simulink model "rlQuadrupedRobot"  (R2020a)
settings: Solver=ode23tb  StartTime=0.0  StopTime=Tf  RelTol=1e-3  EnableMultiTasking=on
undefined symbols (not defined in the file or in its folder): Extr_Data_LinkEndHole, Extr_Data_Mesh, friction_force_max, g, ground, h_final, hip_eq_angle, init_ang_FL, init_ang_FR, init_ang_RL, init_ang_RR, joint, knee_eq_angle, l1, l2, L_back, M, m1, m2, mu_kinetic, mu_static, normal_force_max, pitch_max, q_hip_max, q_hip_min, q_knee_max, q_knee_min, roll_max, Tf, Ts, u_max, v_thres, vx_max, vy_max, vz_max, w_max, X, Y, y_max, y_min, yaw_max, Z, z_max
libraries: sm_lib x145, nesl_utility x87, simulink x12, rllib x1
(part 8 of 8)

== system rlQuadrupedRobot/Quadruped Robot/Leg RL/Contact Forces Model/Sphere to Plane Force/Forces/Ff/SlipVel ==
  wx : Inport
  wy : Inport  Port=2
  vx : Inport  Port=3
  vy : Inport  Port=4
  Fx1 : Constant  Value=sphere_rad
  Math Function : Math  Operator=square  SignedPower=on  SaturateOnIntegerOverflow=on
  Math Function1 : Math  Operator=square  SignedPower=on  SaturateOnIntegerOverflow=on
  Product3 : Product
  Product4 : Product
  Sqrt : Sqrt  SaturateOnIntegerOverflow=on
  Sum1 : Sum  Inputs=|++
  Sum2 : Sum  Inputs=|-+
  Sum3 : Sum  Inputs=|++
  Trigonometric Function : Trigonometry  Operator=atan2
  vabs : Outport  VectorParamsAs1DForOutWhenUnconnected=off
  alpha : Outport  Port=2  VectorParamsAs1DForOutWhenUnconnected=off
  wires:
  wx/1 -> Product3/1
  Product3/1 -> Sum1/1
  wy/1 -> Product4/2
  vx/1 -> Sum2/2
  Fx1/1 -> Product3/2, Product4/1
  vy/1 -> Sum1/2
  Product4/1 -> Sum2/1
  Trigonometric Function/1 -> alpha/1
  Sqrt/1 -> vabs/1
  Sum3/1 -> Sqrt/1
  Math Function/1 -> Sum3/1
  Math Function1/1 -> Sum3/2
  Sum1/1 -> Trigonometric Function/1, Math Function/1  "slipy"
  Sum2/1 -> Trigonometric Function/2, Math Function1/1  "slipx"

== system rlQuadrupedRobot/Quadruped Robot/Leg RL/Contact Forces Model/Sphere to Plane Force/Forces/Force Law/Custom ==
  note: Implement your own custom force law in this subsystem.
      | To use it in the contact force models,
      | set the parameter "Force Law" to "Custom".
  Pen : Inport
  Pen Vel : Inport  Port=2
  Abs : Abs  ZeroCross=off
  Gain1 : Gain  Gain=k_pen  Multiplication=Matrix(K*u)  SaturateOnIntegerOverflow=on  OutDataTypeStr=Inherit: Same as input  ParamDataTypeStr=Inherit: Same as input
  Gain2 : Gain  Gain=-b_penvel  Multiplication=Matrix(K*u)  SaturateOnIntegerOverflow=on  OutDataTypeStr=Inherit: Same as input  ParamDataTypeStr=Inherit: Same as input
  Product : Product  RndMeth=Zero
  Saturation : Saturate  UpperLimit=Inf  LowerLimit=0  ZeroCross=off
  Sign : Signum  ZeroCross=off
  Spr F : Outport  VectorParamsAs1DForOutWhenUnconnected=off
  Damp F : Outport  Port=2  VectorParamsAs1DForOutWhenUnconnected=off
  wires:
  Saturation/1 -> Gain2/1
  Pen/1 -> Sign/1, Gain1/1  "Penetration"
  Abs/1 -> Product/1  "Damping_Force_Enable"
  Product/1 -> Damp F/1  "Damping_Force"
  Sign/1 -> Abs/1
  Pen Vel/1 -> Saturation/1  "Pen Vel"
  Gain2/1 -> Product/2  "Damping_Force"
  Gain1/1 -> Spr F/1  "Stiffness_Force"

== system rlQuadrupedRobot/Quadruped Robot/Leg RL/Contact Forces Model/Sphere to Plane Force/Forces/Force Law/Linear ==
  Pen : Inport
  Pen Vel : Inport  Port=2
  Abs : Abs  ZeroCross=off
  Gain1 : Gain  Gain=k_pen  Multiplication=Matrix(K*u)  SaturateOnIntegerOverflow=on  OutDataTypeStr=Inherit: Same as input  ParamDataTypeStr=Inherit: Same as input
  Gain2 : Gain  Gain=-b_penvel  Multiplication=Matrix(K*u)  SaturateOnIntegerOverflow=on  OutDataTypeStr=Inherit: Same as input  ParamDataTypeStr=Inherit: Same as input
  Product : Product  RndMeth=Zero
  Saturation : Saturate  UpperLimit=Inf  LowerLimit=0  ZeroCross=off
  Sign : Signum  ZeroCross=off
  Spr F : Outport  VectorParamsAs1DForOutWhenUnconnected=off
  Damp F : Outport  Port=2  VectorParamsAs1DForOutWhenUnconnected=off
  wires:
  Saturation/1 -> Gain2/1
  Pen/1 -> Sign/1, Gain1/1  "Penetration"
  Abs/1 -> Product/1  "Damping_Force_Enable"
  Product/1 -> Damp F/1  "Damping_Force"
  Sign/1 -> Abs/1
  Pen Vel/1 -> Saturation/1  "Pen Vel"
  Gain2/1 -> Product/2  "Damping_Force"
  Gain1/1 -> Spr F/1  "Stiffness_Force"

== system rlQuadrupedRobot/Quadruped Robot/Leg RL/Contact Forces Model/Sphere to Plane Force/Forces/Force Law/Nonlinear ==
  Pen : Inport
  Pen Vel : Inport  Port=2
  Constant : Constant  Value=pen_exp
  Gain1 : Gain  Gain=k_pen  Multiplication=Matrix(K*u)  SaturateOnIntegerOverflow=on  OutDataTypeStr=Inherit: Same as input  ParamDataTypeStr=Inherit: Same as input
  Gain2 : Gain  Gain=-b_penvel  Multiplication=Matrix(K*u)  SaturateOnIntegerOverflow=on  OutDataTypeStr=Inherit: Same as input  ParamDataTypeStr=Inherit: Same as input
  Math Function : Math  Operator=pow  SignedPower=on  SaturateOnIntegerOverflow=on
  Product1 : Product  RndMeth=Zero
  Saturation : Saturate  UpperLimit=Inf  LowerLimit=0  ZeroCross=off
  Smoothstep : Subsystem  mask{min_out=0, max_out=1, step_start=0, step_finish=pen_full_damping}
      mask prompts: min_out "Minimum output"; max_out "Maximum output"; step_start "Start Step"; step_finish "Finish Step"
  Spr F : Outport  VectorParamsAs1DForOutWhenUnconnected=off
  Damp F : Outport  Port=2  VectorParamsAs1DForOutWhenUnconnected=off
  wires:
  Saturation/1 -> Gain2/1
  Product1/1 -> Damp F/1
  Smoothstep/1(Out1) -> Product1/1  "Damping_Enable"
  Gain2/1 -> Product1/2  "Damping_Force"
  Constant/1 -> Math Function/2
  Math Function/1 -> Gain1/1
  Pen/1 -> Math Function/1, Smoothstep/1(In1)  "Penetration"
  Pen Vel/1 -> Saturation/1  "Penetration_Velocity"
  Gain1/1 -> Spr F/1  "Stiffness_Force"

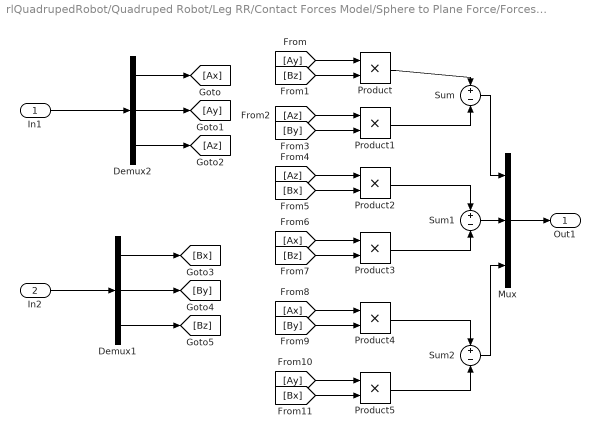
== system rlQuadrupedRobot/Quadruped Robot/Leg RR/Contact Forces Model/Sphere to Plane Force/Forces/Ff/Cross Product ==
  In1 : Inport
  In2 : Inport  Port=2
  Demux1 : Demux  Outputs=3
  Demux2 : Demux  Outputs=3
  Mux : Mux  Inputs=3
  Product{,1..5} (6 alike) : Product
  Sum : Sum  Inputs=+|-
  Sum1 : Sum  Inputs=+|-
  Sum2 : Sum  Inputs=+|-
  Out1 : Outport  VectorParamsAs1DForOutWhenUnconnected=off
  wires:
  In2/1 -> Demux1/1
  Mux/1 -> Out1/1
  Product1/1 -> Sum/2
  Product/1 -> Sum/1
  Product2/1 -> Sum1/1
  Product3/1 -> Sum1/2
  Product4/1 -> Sum2/1
  Product5/1 -> Sum2/2
  Sum1/1 -> Mux/2
  Sum/1 -> Mux/1
  Sum2/1 -> Mux/3
  In1/1 -> Demux2/1
  Demux2/1 -> [Ax]
  Demux2/2 -> [Ay]
  Demux2/3 -> [Az]
  Demux1/1 -> [Bx]
  Demux1/2 -> [By]
  Demux1/3 -> [Bz]
  [Ay] -> Product/1
  [Bz] -> Product/2
  [Az] -> Product1/1
  [By] -> Product1/2
  [Az] -> Product2/1
  [Bx] -> Product2/2
  [Ax] -> Product3/1
  [Bz] -> Product3/2
  [Ax] -> Product4/1
  [By] -> Product4/2
  [Ay] -> Product5/1
  [Bx] -> Product5/2

== system rlQuadrupedRobot/Quadruped Robot/Leg RR/Contact Forces Model/Sphere to Plane Force/Forces/Ff/Friction Law ==
  note: 1) Only subsystems can be added as variant choices at this level
      | 2) Blocks cannot be connected at this level as connectivity is
      | automatically determined at simulation, based on the active variant
  Fn : Inport
  v : Inport  Port=2
  None : Subsystem  VariantControl=None  mask(No Friction){}
      mask help: Friction Force = 0
  "Stick-Slip C " : Subsystem  VariantControl=Stick_Slip_C  mask(Stick-Slip Friction, Continuous){muk=mu_kinetic, mus=mu_static, vth=v_thr}
      mask prompts: muk "Coefficient of Kinetic Friction"; mus "Coefficient of Static Friction"; vth "Velocity Threshold"
      mask help: Implements a continuous stick-slip friction model. Smaller velocity threshold is closer to reality but results in a numerically stiffer system.
  Ff : Outport  VectorParamsAs1DForOutWhenUnconnected=off

== system rlQuadrupedRobot/Quadruped Robot/Leg RR/Contact Forces Model/Sphere to Plane Force/Forces/Ff/SlipVel ==
  wx : Inport
  wy : Inport  Port=2
  vx : Inport  Port=3
  vy : Inport  Port=4
  Fx1 : Constant  Value=sphere_rad
  Math Function : Math  Operator=square  SignedPower=on  SaturateOnIntegerOverflow=on
  Math Function1 : Math  Operator=square  SignedPower=on  SaturateOnIntegerOverflow=on
  Product3 : Product
  Product4 : Product
  Sqrt : Sqrt  SaturateOnIntegerOverflow=on
  Sum1 : Sum  Inputs=|++
  Sum2 : Sum  Inputs=|-+
  Sum3 : Sum  Inputs=|++
  Trigonometric Function : Trigonometry  Operator=atan2
  vabs : Outport  VectorParamsAs1DForOutWhenUnconnected=off
  alpha : Outport  Port=2  VectorParamsAs1DForOutWhenUnconnected=off
  wires:
  wx/1 -> Product3/1
  Product3/1 -> Sum1/1
  wy/1 -> Product4/2
  vx/1 -> Sum2/2
  Fx1/1 -> Product3/2, Product4/1
  vy/1 -> Sum1/2
  Product4/1 -> Sum2/1
  Trigonometric Function/1 -> alpha/1
  Sqrt/1 -> vabs/1
  Sum3/1 -> Sqrt/1
  Math Function/1 -> Sum3/1
  Math Function1/1 -> Sum3/2
  Sum1/1 -> Trigonometric Function/1, Math Function/1  "slipy"
  Sum2/1 -> Trigonometric Function/2, Math Function1/1  "slipx"

== system rlQuadrupedRobot/Quadruped Robot/Leg RR/Contact Forces Model/Sphere to Plane Force/Forces/Force Law/Custom ==
  note: Implement your own custom force law in this subsystem.
      | To use it in the contact force models,
      | set the parameter "Force Law" to "Custom".
  Pen : Inport
  Pen Vel : Inport  Port=2
  Abs : Abs  ZeroCross=off
  Gain1 : Gain  Gain=k_pen  Multiplication=Matrix(K*u)  SaturateOnIntegerOverflow=on  OutDataTypeStr=Inherit: Same as input  ParamDataTypeStr=Inherit: Same as input
  Gain2 : Gain  Gain=-b_penvel  Multiplication=Matrix(K*u)  SaturateOnIntegerOverflow=on  OutDataTypeStr=Inherit: Same as input  ParamDataTypeStr=Inherit: Same as input
  Product : Product  RndMeth=Zero
  Saturation : Saturate  UpperLimit=Inf  LowerLimit=0  ZeroCross=off
  Sign : Signum  ZeroCross=off
  Spr F : Outport  VectorParamsAs1DForOutWhenUnconnected=off
  Damp F : Outport  Port=2  VectorParamsAs1DForOutWhenUnconnected=off
  wires:
  Saturation/1 -> Gain2/1
  Pen/1 -> Sign/1, Gain1/1  "Penetration"
  Abs/1 -> Product/1  "Damping_Force_Enable"
  Product/1 -> Damp F/1  "Damping_Force"
  Sign/1 -> Abs/1
  Pen Vel/1 -> Saturation/1  "Pen Vel"
  Gain2/1 -> Product/2  "Damping_Force"
  Gain1/1 -> Spr F/1  "Stiffness_Force"

== system rlQuadrupedRobot/Quadruped Robot/Leg RR/Contact Forces Model/Sphere to Plane Force/Forces/Force Law/Linear ==
  Pen : Inport
  Pen Vel : Inport  Port=2
  Abs : Abs  ZeroCross=off
  Gain1 : Gain  Gain=k_pen  Multiplication=Matrix(K*u)  SaturateOnIntegerOverflow=on  OutDataTypeStr=Inherit: Same as input  ParamDataTypeStr=Inherit: Same as input
  Gain2 : Gain  Gain=-b_penvel  Multiplication=Matrix(K*u)  SaturateOnIntegerOverflow=on  OutDataTypeStr=Inherit: Same as input  ParamDataTypeStr=Inherit: Same as input
  Product : Product  RndMeth=Zero
  Saturation : Saturate  UpperLimit=Inf  LowerLimit=0  ZeroCross=off
  Sign : Signum  ZeroCross=off
  Spr F : Outport  VectorParamsAs1DForOutWhenUnconnected=off
  Damp F : Outport  Port=2  VectorParamsAs1DForOutWhenUnconnected=off
  wires:
  Saturation/1 -> Gain2/1
  Pen/1 -> Sign/1, Gain1/1  "Penetration"
  Abs/1 -> Product/1  "Damping_Force_Enable"
  Product/1 -> Damp F/1  "Damping_Force"
  Sign/1 -> Abs/1
  Pen Vel/1 -> Saturation/1  "Pen Vel"
  Gain2/1 -> Product/2  "Damping_Force"
  Gain1/1 -> Spr F/1  "Stiffness_Force"

== system rlQuadrupedRobot/Quadruped Robot/Leg RR/Contact Forces Model/Sphere to Plane Force/Forces/Force Law/Nonlinear ==
  Pen : Inport
  Pen Vel : Inport  Port=2
  Constant : Constant  Value=pen_exp
  Gain1 : Gain  Gain=k_pen  Multiplication=Matrix(K*u)  SaturateOnIntegerOverflow=on  OutDataTypeStr=Inherit: Same as input  ParamDataTypeStr=Inherit: Same as input
  Gain2 : Gain  Gain=-b_penvel  Multiplication=Matrix(K*u)  SaturateOnIntegerOverflow=on  OutDataTypeStr=Inherit: Same as input  ParamDataTypeStr=Inherit: Same as input
  Math Function : Math  Operator=pow  SignedPower=on  SaturateOnIntegerOverflow=on
  Product1 : Product  RndMeth=Zero
  Saturation : Saturate  UpperLimit=Inf  LowerLimit=0  ZeroCross=off
  Smoothstep : Subsystem  mask{min_out=0, max_out=1, step_start=0, step_finish=pen_full_damping}
      mask prompts: min_out "Minimum output"; max_out "Maximum output"; step_start "Start Step"; step_finish "Finish Step"
  Spr F : Outport  VectorParamsAs1DForOutWhenUnconnected=off
  Damp F : Outport  Port=2  VectorParamsAs1DForOutWhenUnconnected=off
  wires:
  Saturation/1 -> Gain2/1
  Product1/1 -> Damp F/1
  Smoothstep/1(Out1) -> Product1/1  "Damping_Enable"
  Gain2/1 -> Product1/2  "Damping_Force"
  Constant/1 -> Math Function/2
  Math Function/1 -> Gain1/1
  Pen/1 -> Math Function/1, Smoothstep/1(In1)  "Penetration"
  Pen Vel/1 -> Saturation/1  "Penetration_Velocity"
  Gain1/1 -> Spr F/1  "Stiffness_Force"

== system rlQuadrupedRobot/Quadruped Robot/Leg FL/Contact Forces Model/Sphere to Plane Force/Forces/Ff/Friction Law/None ==
  Fn : Inport
  v : Inport  Port=2
  Constant : Constant  Value=0
  Terminator : Terminator
  Terminator1 : Terminator
  Ff : Outport  VectorParamsAs1DForOutWhenUnconnected=off
  wires:
  Constant/1 -> Ff/1  "Friction_Force"
  v/1 -> Terminator/1  "Velocity"
  Fn/1 -> Terminator1/1  "Normal_Force"

== system rlQuadrupedRobot/Quadruped Robot/Leg FL/Contact Forces Model/Sphere to Plane Force/Forces/Ff/Friction Law/Stick-Slip C  ==
  Fn : Inport
  v : Inport  Port=2
  Coefficient of Friction vs Velocity : Lookup_n-D  NumberOfTableDimensions=1  BreakpointsForDimension1=[-3 -1.5 -1 1 1.5 3]*vth  Table="[-muk -muk -mus mus  muk muk]"  InternalRulePriority=Speed  InputSameDT=on
  Gain2 : Gain  Multiplication=Matrix(K*u)  SaturateOnIntegerOverflow=on  OutDataTypeStr=Inherit: Same as input  ParamDataTypeStr=Inherit: Same as input
  Product : Product  RndMeth=Zero
  Ff : Outport  VectorParamsAs1DForOutWhenUnconnected=off
  wires:
  Fn/1 -> Product/2  "Normal_Force"
  Coefficient of Friction vs Velocity/1 -> Product/1
  v/1 -> Coefficient of Friction vs Velocity/1  "Velocity"
  Product/1 -> Gain2/1
  Gain2/1 -> Ff/1  "Friction_Force"

== system rlQuadrupedRobot/Quadruped Robot/Leg FL/Contact Forces Model/Sphere to Plane Force/Forces/Force Law/Nonlinear/Smoothstep ==
  In1 : Inport
  Clamp : Saturate  UpperLimit=step_finish  LowerLimit=step_start
  Constant : Constant  Value=3
  Divide : Product  Inputs=*/
  Divide1 : Product  Inputs=****
  Gain : Gain  Gain=2
  Subtract : Sum  Inputs=+-
  Subtract1 : Sum  Inputs=-+
  Subtract2 : Sum
  Subtract3 : Sum  Inputs=+-
  Subtract4 : Sum  Inputs=+-
  max out : Constant  Value=max_out
  min out : Constant  Value=min_out
  step finish : Constant  Value=step_finish
  step start : Constant  Value=step_start
  Out1 : Outport  VectorParamsAs1DForOutWhenUnconnected=off
  wires:
  step start/1 -> Subtract1/1, Subtract/2
  In1/1 -> Clamp/1
  Subtract1/1 -> Divide/2
  Divide/1 -> Gain/1, Divide1/2, Divide1/3
  Subtract/1 -> Divide/1
  Subtract2/1 -> Out1/1
  Constant/1 -> Subtract4/1
  min out/1 -> Subtract2/2, Subtract3/2
  max out/1 -> Subtract3/1
  Clamp/1 -> Subtract/1
  step finish/1 -> Subtract1/2
  Divide1/1 -> Subtract2/1
  Gain/1 -> Subtract4/2
  Subtract4/1 -> Divide1/1
  Subtract3/1 -> Divide1/4

== system rlQuadrupedRobot/Quadruped Robot/Leg FR/Contact Forces Model/Sphere to Plane Force/Forces/Ff/Friction Law/None ==
  Fn : Inport
  v : Inport  Port=2
  Constant : Constant  Value=0
  Terminator : Terminator
  Terminator1 : Terminator
  Ff : Outport  VectorParamsAs1DForOutWhenUnconnected=off
  wires:
  Constant/1 -> Ff/1  "Friction_Force"
  v/1 -> Terminator/1  "Velocity"
  Fn/1 -> Terminator1/1  "Normal_Force"

== system rlQuadrupedRobot/Quadruped Robot/Leg FR/Contact Forces Model/Sphere to Plane Force/Forces/Ff/Friction Law/Stick-Slip C  ==
  Fn : Inport
  v : Inport  Port=2
  Coefficient of Friction vs Velocity : Lookup_n-D  NumberOfTableDimensions=1  BreakpointsForDimension1=[-3 -1.5 -1 1 1.5 3]*vth  Table="[-muk -muk -mus mus  muk muk]"  InternalRulePriority=Speed  InputSameDT=on
  Gain2 : Gain  Multiplication=Matrix(K*u)  SaturateOnIntegerOverflow=on  OutDataTypeStr=Inherit: Same as input  ParamDataTypeStr=Inherit: Same as input
  Product : Product  RndMeth=Zero
  Ff : Outport  VectorParamsAs1DForOutWhenUnconnected=off
  wires:
  Fn/1 -> Product/2  "Normal_Force"
  Coefficient of Friction vs Velocity/1 -> Product/1
  v/1 -> Coefficient of Friction vs Velocity/1  "Velocity"
  Product/1 -> Gain2/1
  Gain2/1 -> Ff/1  "Friction_Force"

== system rlQuadrupedRobot/Quadruped Robot/Leg FR/Contact Forces Model/Sphere to Plane Force/Forces/Force Law/Nonlinear/Smoothstep ==
  In1 : Inport
  Clamp : Saturate  UpperLimit=step_finish  LowerLimit=step_start
  Constant : Constant  Value=3
  Divide : Product  Inputs=*/
  Divide1 : Product  Inputs=****
  Gain : Gain  Gain=2
  Subtract : Sum  Inputs=+-
  Subtract1 : Sum  Inputs=-+
  Subtract2 : Sum
  Subtract3 : Sum  Inputs=+-
  Subtract4 : Sum  Inputs=+-
  max out : Constant  Value=max_out
  min out : Constant  Value=min_out
  step finish : Constant  Value=step_finish
  step start : Constant  Value=step_start
  Out1 : Outport  VectorParamsAs1DForOutWhenUnconnected=off
  wires:
  step start/1 -> Subtract1/1, Subtract/2
  In1/1 -> Clamp/1
  Subtract1/1 -> Divide/2
  Divide/1 -> Gain/1, Divide1/2, Divide1/3
  Subtract/1 -> Divide/1
  Subtract2/1 -> Out1/1
  Constant/1 -> Subtract4/1
  min out/1 -> Subtract2/2, Subtract3/2
  max out/1 -> Subtract3/1
  Clamp/1 -> Subtract/1
  step finish/1 -> Subtract1/2
  Divide1/1 -> Subtract2/1
  Gain/1 -> Subtract4/2
  Subtract4/1 -> Divide1/1
  Subtract3/1 -> Divide1/4

== system rlQuadrupedRobot/Quadruped Robot/Leg RL/Contact Forces Model/Sphere to Plane Force/Forces/Ff/Friction Law/None ==
  Fn : Inport
  v : Inport  Port=2
  Constant : Constant  Value=0
  Terminator : Terminator
  Terminator1 : Terminator
  Ff : Outport  VectorParamsAs1DForOutWhenUnconnected=off
  wires:
  Constant/1 -> Ff/1  "Friction_Force"
  v/1 -> Terminator/1  "Velocity"
  Fn/1 -> Terminator1/1  "Normal_Force"

== system rlQuadrupedRobot/Quadruped Robot/Leg RL/Contact Forces Model/Sphere to Plane Force/Forces/Ff/Friction Law/Stick-Slip C  ==
  Fn : Inport
  v : Inport  Port=2
  Coefficient of Friction vs Velocity : Lookup_n-D  NumberOfTableDimensions=1  BreakpointsForDimension1=[-3 -1.5 -1 1 1.5 3]*vth  Table="[-muk -muk -mus mus  muk muk]"  InternalRulePriority=Speed  InputSameDT=on
  Gain2 : Gain  Multiplication=Matrix(K*u)  SaturateOnIntegerOverflow=on  OutDataTypeStr=Inherit: Same as input  ParamDataTypeStr=Inherit: Same as input
  Product : Product  RndMeth=Zero
  Ff : Outport  VectorParamsAs1DForOutWhenUnconnected=off
  wires:
  Fn/1 -> Product/2  "Normal_Force"
  Coefficient of Friction vs Velocity/1 -> Product/1
  v/1 -> Coefficient of Friction vs Velocity/1  "Velocity"
  Product/1 -> Gain2/1
  Gain2/1 -> Ff/1  "Friction_Force"

== system rlQuadrupedRobot/Quadruped Robot/Leg RL/Contact Forces Model/Sphere to Plane Force/Forces/Force Law/Nonlinear/Smoothstep ==
  In1 : Inport
  Clamp : Saturate  UpperLimit=step_finish  LowerLimit=step_start
  Constant : Constant  Value=3
  Divide : Product  Inputs=*/
  Divide1 : Product  Inputs=****
  Gain : Gain  Gain=2
  Subtract : Sum  Inputs=+-
  Subtract1 : Sum  Inputs=-+
  Subtract2 : Sum
  Subtract3 : Sum  Inputs=+-
  Subtract4 : Sum  Inputs=+-
  max out : Constant  Value=max_out
  min out : Constant  Value=min_out
  step finish : Constant  Value=step_finish
  step start : Constant  Value=step_start
  Out1 : Outport  VectorParamsAs1DForOutWhenUnconnected=off
  wires:
  step start/1 -> Subtract1/1, Subtract/2
  In1/1 -> Clamp/1
  Subtract1/1 -> Divide/2
  Divide/1 -> Gain/1, Divide1/2, Divide1/3
  Subtract/1 -> Divide/1
  Subtract2/1 -> Out1/1
  Constant/1 -> Subtract4/1
  min out/1 -> Subtract2/2, Subtract3/2
  max out/1 -> Subtract3/1
  Clamp/1 -> Subtract/1
  step finish/1 -> Subtract1/2
  Divide1/1 -> Subtract2/1
  Gain/1 -> Subtract4/2
  Subtract4/1 -> Divide1/1
  Subtract3/1 -> Divide1/4

== system rlQuadrupedRobot/Quadruped Robot/Leg RR/Contact Forces Model/Sphere to Plane Force/Forces/Ff/Friction Law/None ==
  Fn : Inport
  v : Inport  Port=2
  Constant : Constant  Value=0
  Terminator : Terminator
  Terminator1 : Terminator
  Ff : Outport  VectorParamsAs1DForOutWhenUnconnected=off
  wires:
  Constant/1 -> Ff/1  "Friction_Force"
  v/1 -> Terminator/1  "Velocity"
  Fn/1 -> Terminator1/1  "Normal_Force"

== system rlQuadrupedRobot/Quadruped Robot/Leg RR/Contact Forces Model/Sphere to Plane Force/Forces/Ff/Friction Law/Stick-Slip C  ==
  Fn : Inport
  v : Inport  Port=2
  Coefficient of Friction vs Velocity : Lookup_n-D  NumberOfTableDimensions=1  BreakpointsForDimension1=[-3 -1.5 -1 1 1.5 3]*vth  Table="[-muk -muk -mus mus  muk muk]"  InternalRulePriority=Speed  InputSameDT=on
  Gain2 : Gain  Multiplication=Matrix(K*u)  SaturateOnIntegerOverflow=on  OutDataTypeStr=Inherit: Same as input  ParamDataTypeStr=Inherit: Same as input
  Product : Product  RndMeth=Zero
  Ff : Outport  VectorParamsAs1DForOutWhenUnconnected=off
  wires:
  Fn/1 -> Product/2  "Normal_Force"
  Coefficient of Friction vs Velocity/1 -> Product/1
  v/1 -> Coefficient of Friction vs Velocity/1  "Velocity"
  Product/1 -> Gain2/1
  Gain2/1 -> Ff/1  "Friction_Force"

== system rlQuadrupedRobot/Quadruped Robot/Leg RR/Contact Forces Model/Sphere to Plane Force/Forces/Force Law/Nonlinear/Smoothstep ==
  In1 : Inport
  Clamp : Saturate  UpperLimit=step_finish  LowerLimit=step_start
  Constant : Constant  Value=3
  Divide : Product  Inputs=*/
  Divide1 : Product  Inputs=****
  Gain : Gain  Gain=2
  Subtract : Sum  Inputs=+-
  Subtract1 : Sum  Inputs=-+
  Subtract2 : Sum
  Subtract3 : Sum  Inputs=+-
  Subtract4 : Sum  Inputs=+-
  max out : Constant  Value=max_out
  min out : Constant  Value=min_out
  step finish : Constant  Value=step_finish
  step start : Constant  Value=step_start
  Out1 : Outport  VectorParamsAs1DForOutWhenUnconnected=off
  wires:
  step start/1 -> Subtract1/1, Subtract/2
  In1/1 -> Clamp/1
  Subtract1/1 -> Divide/2
  Divide/1 -> Gain/1, Divide1/2, Divide1/3
  Subtract/1 -> Divide/1
  Subtract2/1 -> Out1/1
  Constant/1 -> Subtract4/1
  min out/1 -> Subtract2/2, Subtract3/2
  max out/1 -> Subtract3/1
  Clamp/1 -> Subtract/1
  step finish/1 -> Subtract1/2
  Divide1/1 -> Subtract2/1
  Gain/1 -> Subtract4/2
  Subtract4/1 -> Divide1/1
  Subtract3/1 -> Divide1/4

== matlab function rlQuadrupedRobot/Check If Done/MATLAB Function ==
  data: q input; R output
function R = quatToRotM(q)
% Quaternion to Rotation matrix conversion
% Source: https://en.wikipedia.org/wiki/Quaternions_and_spatial_rotation#Quaternion-derived_rotation_matrix

% Normalize the quaternions
q = bsxfun(@times, q, 1./sqrt(sum(q.^2,1)));

q0 = q(1);
q1 = q(2);
q2 = q(3);
q3 = q(4);

r11 = 1 - 2*(q2^2+q3^2);
r12 = 2*(q1*q2-q0*q3);
r13 = 2*(q0*q2+q1*q3);
r21 = 2*(q1*q2+q0*q3);
r22 = 1 - 2*(q1^2+q3^2);
r23 = 2*(q2*q3-q0*q1);
r31 = 2*(q1*q3-q0*q2);
r32 = 2*(q0*q1+q2*q3);
r33 = 1 - 2*(q1^2+q2^2);

R = [r11 r12 r13; r21 r22 r23; r31 r32 r33];

== matlab function rlQuadrupedRobot/Reward/MATLAB Function ==
  data: q input; e output
function e = quatToEuler(q)

% Normalize the quaternions
q = bsxfun(@times, q, 1./sqrt(sum(q.^2,1)));

qw = q(1);
qx = q(2);
qy = q(3);
qz = q(4);

% Pre-allocate output
%e = zeros(3, 1, 'like', q);

aSinInput = -2*(qx.*qz-qw.*qy);
aSinInput(aSinInput > 1) = 1;
aSinInput(aSinInput < -1) = -1;

e = [ atan2( 2*(qx.*qy+qw.*qz), qw.^2 + qx.^2 - qy.^2 - qz.^2 ); ...
    asin( aSinInput ); ...
    atan2( 2*(qy.*qz+qw.*qx), qw.^2 - qx.^2 - qy.^2 + qz.^2 )];

% roll = atan2(2*(q0*q1+q2*q3),(1-2*(q1^2+q2^2)));  %phi
% yaw = asin(2*(q0*q2-q3*q1));
% pitch = atan2(2*(q0*q3+q1*q2),(1-2*(q2^2+q3^2)));
% 
% e = [pitch; yaw; roll];  % ZYX
